simulink model "pend_non_linear_up"  (R2018b)
settings: Solver=ode15s  StartTime=0.0  StopTime=10  MaxStep=0.2  RelTol=1e-6
values from neighbouring files (symbols this model uses):
  Jm = 3.1e-7    (= 3.1e-07)    [main.m]    (also in pend.m)
  Jp = 1774.274e-6    (= 0.001774274)    [main.m]    (also in pend.m)
  Kf = 7.44e-3    (= 0.00744)    [main.m]    (also in pend.m)
  La = 35e-6    (= 3.5e-05)    [main.m]    (also in pend.m)
  lb = 141.451e-3    (= 0.141451)    [main.m]    (also in pend.m)
  M = 879.5e-3    (= 0.8795)    [main.m]    (also in pend.m)
  m = 135.4e-3    (= 0.1354)    [main.m]    (also in pend.m)
  r = 0.01    [main.m]    (also in pend.m)
  Ra = 3.92    [main.m]    (also in pend.m)
  Rg = (13.55+11.04)/4    (= 6.1475)    [main.m]    (also in pend.m)
  rt = 0.01    [main.m]    (also in pend.m)
  Va = 0    [main.m]    (also in pend.m = 1)
settings Model: Creator=Tulio  LastModifiedBy=Tulio

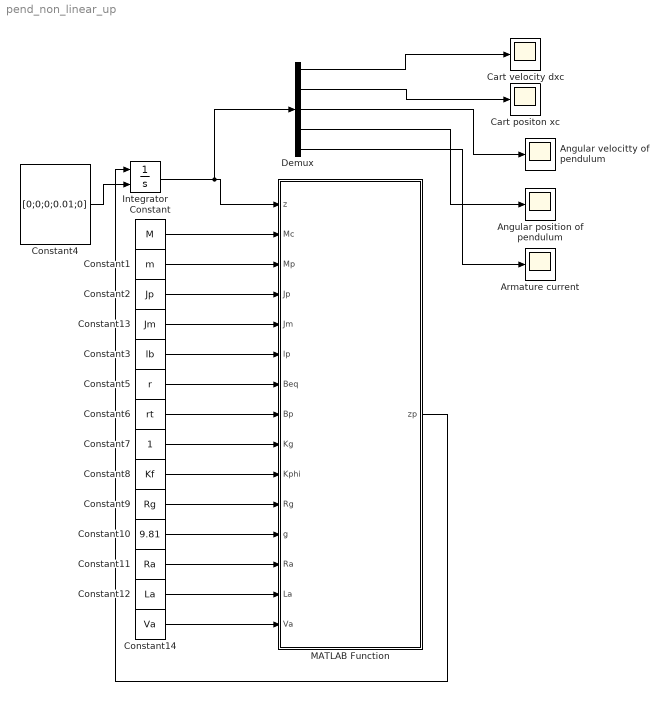
== system pend_non_linear_up ==
  Angular position of pendulum : Scope
  "Angular velocitty of pendulum " : Scope
  Armature current : Scope
  Cart positon xc : Scope
  Cart velocity dxc : Scope
  Constant : Constant  Value=M
  Constant1 : Constant  Value=m
  Constant10 : Constant  Value=9.81
  Constant11 : Constant  Value=Ra
  Constant12 : Constant  Value=La
  Constant13 : Constant  Value=Jm
  Constant14 : Constant  Value=Va
  Constant2 : Constant  Value=Jp
  Constant3 : Constant  Value=lb
  Constant4 : Constant  Value=[0;0;0;0.01;0]
  Constant5 : Constant  Value=r
  Constant6 : Constant  Value=rt
  Constant7 : Constant
  Constant8 : Constant  Value=Kf
  Constant9 : Constant  Value=Rg
  Demux : Demux  Outputs=5
  Integrator : Integrator  InitialConditionSource=external
  MATLAB Function : MATLAB Function  TreatAsAtomicUnit=on
  wires:
  MATLAB Function/1(zp) -> Integrator/1
  Integrator/1 -> Demux/1, MATLAB Function/1(z)
  Constant/1 -> MATLAB Function/2(Mc)
  Constant1/1 -> MATLAB Function/3(Mp)
  Constant2/1 -> MATLAB Function/4(Jp)
  Constant3/1 -> MATLAB Function/6(lp)
  Constant4/1 -> Integrator/2
  Constant5/1 -> MATLAB Function/7(Beq)
  Constant6/1 -> MATLAB Function/8(Bp)
  Constant7/1 -> MATLAB Function/9(Kg)
  Constant8/1 -> MATLAB Function/10(Kphi)
  Constant9/1 -> MATLAB Function/11(Rg)
  Constant10/1 -> MATLAB Function/12(g)
  Constant11/1 -> MATLAB Function/13(Ra)
  Constant12/1 -> MATLAB Function/14(La)
  Constant13/1 -> MATLAB Function/5(Jm)
  Constant14/1 -> MATLAB Function/15(Va)
  Demux/2 -> Cart positon xc/1
  Demux/4 -> Angular position of pendulum/1
  Demux/1 -> Cart velocity dxc/1
  Demux/3 -> "Angular velocitty of pendulum "/1
  Demux/5 -> Armature current/1

== matlab function pend_non_linear_up/MATLAB Function ==
  data: z input; zp output; Mc input; Mp input; Jp input; Jm input; lp input; Beq input; Bp input; Kg input; Kphi input; Rg input; g input; Ra input; La input; Va input
function zp = fcn(z,Mc,Mp,Jp,Jm,lp,Beq,Bp,Kg,Kphi,Rg,g,Ra,La,Va)
% z = [xcp xc thetap theta Ia]
xcp = z(1); xc = z(2); thetap = z(3); theta = z(4); Ia = z(5);
AA = [Mc+Mp+Jm*(Kg/Rg)^2,0,Mp*lp*cos(theta),0,0;
      0,1,0,0,0;
      Mp*lp*cos(theta),0,Jp+Mp*lp^2,0,0;
      0,0,0,1,0;
      0,0,0,0,1];
F = [Mp*lp*sin(theta)*thetap^2 - Beq*xcp + Kg*Kphi/Rg*Ia;
     xcp;
     -Bp*thetap + Mp*lp*g*sin(theta);
     thetap;
     -Ra/La*Ia - Kg*Kphi/Rg/La*xcp;
    ];
B = [0;0;0;0;1/La];

zp = inv(AA)*F+B*Va;

end
